simulink model "FULLORDERUNKNOW"  (R2015b)
settings: Solver=VariableStepAuto  StartTime=0.0  StopTime=10.0  RelTol=1e-3
values from neighbouring files (symbols this model uses):
  A = [-1 -1 0;-1 0 0;0 -1 -1]    [FULLORDERUNKNOWN.m]    (also in OBSERVER.m = [0 20.6;1 0]; functional.m = [-10 2 0 1 0; 1 -1 0 0 1;1 0 -5 3 4; -3 1 1 -8 3; -2 -4 0 2 ; lmi.m = [-10 2 0 1 0; 1 -1 0 0 1;1 0 -5 3 4; -3 1 1 -8 3; -2 -4 0 2 ; reduced_observer.m = [1 0 -2 2 0 0 -8 -6 -2;0 -1 3 18 41 -10 -19 -28 4; 1 2 3 4 4)
  B = [1;2;3]    [FULLORDERUNKNOWN.m]    (also in OBSERVER.m = [0;1]; functional.m = [1;2;3;4;5]; lmi.m = [1;2;3;4;5]; reduced_observer.m = [1;2;3;4;5;6;7;8;9])
  C = [1 0 0;0 0 1]    [FULLORDERUNKNOWN.m]    (also in OBSERVER.m = [0 1]; functional.m = [1 0 0 0 0;0 1 0 0 0]; lmi.m = [1 0 0 0 0;0 1 0 0 0]; reduced_observer.m = [1 0 0 0 0 0 0 0 0;0 1 0 0 0 0 0 0 0; 0 0 1 0 0 0 0 0 0])
  E = W*pinv(C*W)+Z*(eye(2)-(C*W)*(pinv(C*W)))    [FULLORDERUNKNOWN.m]
  H = Y*B    [FULLORDERUNKNOWN.m]    (also in reduced_observer.m = B2-L*B1)
  J = L+N*E    [FULLORDERUNKNOWN.m]
  k = place(A,B,e)    [FULLORDERUNKNOWN.m]    (also in OBSERVER.m; functional.m = cell(Y,1); reduced_observer.m)
  N = Y*A-L*C    [FULLORDERUNKNOWN.m]    (also in lmi.m = dec2mat(lmisys,dvar,N))
  W = [-1;0;0]    [FULLORDERUNKNOWN.m]
settings Model: Creator=deepika  LastModifiedBy=deepika

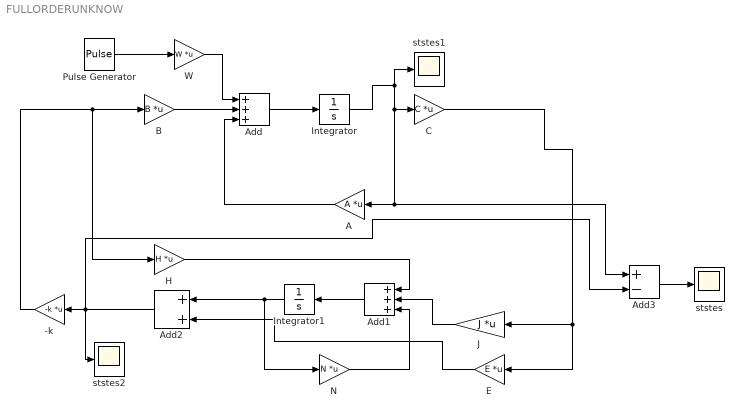
== system FULLORDERUNKNOW ==
  " ststes" : Scope
  " ststes1" : Scope
  " ststes2" : Scope
  -k : Gain  Gain=-k  Multiplication=Matrix(K*u)
  A : Gain  Gain=A  Multiplication=Matrix(K*u)
  Add : Sum  Inputs=+++
  Add1 : Sum  Inputs=+++
  Add2 : Sum
  Add3 : Sum  Inputs=+-
  B : Gain  Gain=B  Multiplication=Matrix(K*u)
  C : Gain  Gain=C  Multiplication=Matrix(K*u)
  E : Gain  Gain=E  Multiplication=Matrix(K*u)
  H : Gain  Gain=H  Multiplication=Matrix(K*u)
  Integrator : Integrator
  Integrator1 : Integrator
  J : Gain  Gain=J  Multiplication=Matrix(K*u)
  N : Gain  Gain=N  Multiplication=Matrix(K*u)
  Pulse Generator : DiscretePulseGenerator  PulseType=Time based  Period=.05  PulseWidth=50
  W : Gain  Gain=W  Multiplication=Matrix(K*u)
  wires:
  B/1 -> Add/2
  Add/1 -> Integrator/1
  Integrator/1 -> Add3/1, A/1, C/1, " ststes1"/1
  A/1 -> Add/3
  C/1 -> E/1, J/1
  J/1 -> Add1/2
  Add1/1 -> Integrator1/1
  Integrator1/1 -> Add2/1, N/1
  N/1 -> Add1/3
  H/1 -> Add1/1
  E/1 -> Add2/2
  Add2/1 -> " ststes2"/1, Add3/2, -k/1
  -k/1 -> H/1, B/1
  W/1 -> Add/1
  Pulse Generator/1 -> W/1
  Add3/1 -> " ststes"/1
